simulink subsystem "AC_bypass_pipe_3zone_R2024a"  (R2024a)
settings: Solver=VariableStepAuto  StartTime=0.0  StopTime=10.0  RelTol=1e-3
undefined symbols (not defined in the file or in its folder): Ambient_temp
libraries: fl_lib x2, nesl_utility x2, SimscapeFluids_lib x1
settings Model: Creator=MW  LastModifiedBy=hc21562

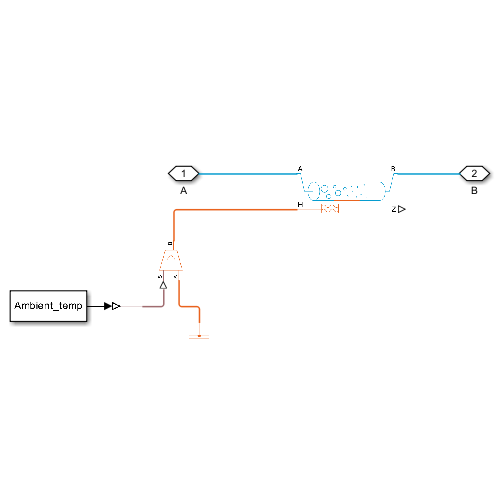
[thumbnail: Simulink's stored preview of the top-level diagram]
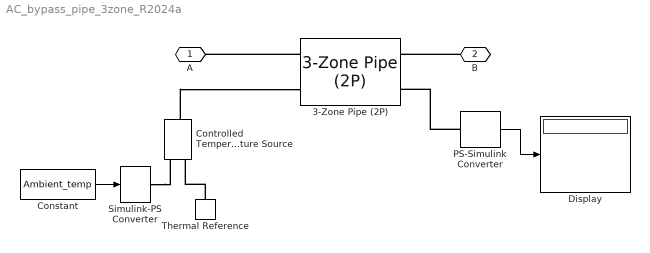
== system AC_bypass_pipe_3zone_R2024a ==
  3-Zone Pipe (2P) : SimscapeFluids_lib/Two-Phase Fluid/Pipes & Fittings/3-Zone Pipe (2P)  length=AC_bypass_pipe_length m  area=AC_bypass_line_port_inner_area m^2  Dh=AC_bypass_line_port_inner_diameter m  elevation_gain=AC_bypass_pipe_length m  g=9.81 m/s^2  length_add=0.1 m  roughness=15e-6 m  Re_lam=Re_laminar_max  Re_tur=Re_turbulent_min  shape_factor=64  hc_ext=pipe_thermal_conductivity W/(K*m^2)  wall_thickness=wall_thickness m  k_wall=steel_conductivity W/(K*m)  c_wall=steel_heat_capacity J/(K*kg)  rho_wall=steel_density kg/m^3  fin_ratio_ext=0  eta_fin_ext=0.5  fin_ratio_int=0  eta_fin_int=0.5  heat_coeff_spec=fluids.two_phase_fluid.pipes_fittings.enum.HeatCoeffSpec.GnielinskiCavalliniZecchin  colburn_coeff_liq=[.023, .8, .33]  colburn_coeff_mix=[.05, .8, .33]  colburn_coeff_vap=[.023, .8, .33]  Nu_lam=3.66  energy_spec=foundation.enum.energy_spec.temperature  p_init=initial_hose_p bar  T_init=Initial_temp K  x_init=0.5  alpha_init=0.5  h_init=1500 kJ/kg  u_init=1500 kJ/kg
      settings: InternalSimscapePortConfiguration="{\"Bottom\":[],\"Left\":[{\"id\":\"A\",\"label\":\"A\",\"type\":\"foundation.two_phase_fluid.two_phase_fluid\"},{\"id\":\"H\",\"label\":\"H\",\"type\":\"foundation.thermal.thermal\"}],\"Right\":[{\"id\":\"B\",\"label\":\"B\",\"type\":\"foundation.two_phase_fluid.two_phase_fluid\"},{\"id\":\"Z\",\"label\":\"Z\",\"type\":\"output\"}],\"Top\":[]}"
  Constant : Constant  Value=Ambient_temp
  Controlled Temperature Source : fl_lib/Thermal/Thermal Sources/Controlled Temperature Source
  Display : Display
  PS-Simulink Converter : nesl_utility/PS-Simulink Converter  PhysicalDomain=network_engine_domain  SubClassName=ps_output  LeftPortType=input  RightPortType=output  PseudoPeriodic=off  Frequencies=[]  VectorFormat=inherit  Unit=inherit  AffineConversion=off
  Simulink-PS Converter : nesl_utility/Simulink-PS Converter  PhysicalDomain=network_engine_domain  SubClassName=ps_input  LeftPortType=input  RightPortType=output  PseudoPeriodic=off  Frequencies=[]  NoiseDistribution=none  NoiseParameters=[]  Unit=1  AffineConversion=off  FilteringAndDerivatives=zero  SimscapeFilterOrder=1  InputFilterTimeConstant=0.001  UdotUserProvided=1
  Thermal Reference : fl_lib/Thermal/Thermal Elements/Thermal Reference
  A : PMIOPort  Side=Left
  B : PMIOPort  Port=2  Side=Right
  wires:
  Constant/1 -> Simulink-PS Converter/1
  PS-Simulink Converter/1 -> Display/1
  connections:
  Controlled Temperature Source/LConn1 -- 3-Zone Pipe (2P)/LConn2
  B/RConn1 -- 3-Zone Pipe (2P)/RConn1
  Thermal Reference/LConn1 -- Controlled Temperature Source/RConn2
  Simulink-PS Converter/RConn1 -- Controlled Temperature Source/RConn1
  3-Zone Pipe (2P)/LConn1 -- A/RConn1
  PS-Simulink Converter/LConn1 -- 3-Zone Pipe (2P)/RConn2
